simulink model "Impulse_response_system"  (R2022b)
settings: Solver=VariableStepAuto  StartTime=0  StopTime=Tend  FixedStep=0.01  MaxStep=0.1  RelTol=1  AbsTol=1
values from neighbouring files (symbols this model uses):
  I_conversione = Paz.I_conversione    [Glucose_insuline_response.m]    (also in Insulin_controller.m; patient_generator.m = conc_insulina_litro_plasma_Kg)
  IIRb = u(3)    [G_I_Model.m]    (also in Glucose_insuline_response.m = Paz.IIRb; Insulin_controller.m = Paz.IIRb; patient_generator.m = Bolus_die/2)
  Ipb = Paz.Ipb    [Glucose_insuline_response.m]    (also in patient_generator.m = IIRb/(m2+m4 -(m1*m2)/(m1+m3)))
  Pasti = [0,0,0]    [Glucose_insuline_response.m]    (also in Insulin_controller.m = Pasti0+0.2*(-1+2*rand(3,1)).*Pasti0; patient_generator.m = Pasti0)
  Tpasti = Tpasti0    [Glucose_insuline_response.m]    (also in Insulin_controller.m = Tpasti0+delta_T)
  x0 = y(end,1:13)'    [Glucose_insuline_response.m]    (also in Insulin_controller.m; patient_generator.m = [Gp Gt Il Ip I1 Id Qsto1 Qsto2 Qgut X Isc1 Isc2 Dstato])
undefined symbols (not defined in the file or in its folder): Paz
settings Model: Creator=federico  LastModifiedBy=federico
settings SolverCC: MaxConsecutiveMinStep=auto
settings DataIOCC: SaveFormat=Array  SignalLoggingSaveFormat=ModelDataLogs  ReturnWorkspaceOutputs=off
settings OptimizationCC: BlockReduction=off  BooleanDataType=off  InitFltsAndDblsToZero=on  LifeSpan=inf
settings DebuggingCC: SaveWithParameterizedLinksMsg=none  UnderspecifiedInitializationDetection=Classic  MergeDetectMultiDrivingBlocksExec=none  SignalResolutionControl=TryResolveAllWithWarning  MultiTaskDSMMsg=warning  MultiTaskCondExecSysMsg=none  UnconnectedInputMsg=warning  UnconnectedOutputMsg=warning  UnconnectedLineMsg=warning  SFUnexpectedBacktrackingDiag=warning  SFNoUnconditionalDefaultTransitionDiag=warning  SFExecutionAtInitializationDiag=none  SFMachineParentedDataDiag=warning  ArithmeticOperatorsInVariantConditions=warning
settings HardwareCC: ProdBitPerPointer=32  ProdBitPerSizeT=32  ProdBitPerPtrDiffT=32  ProdLargestAtomicFloat=None  ProdIntDivRoundTo=Undefined  ProdEndianess=Unspecified  ProdWordSize=32  ProdHWDeviceType=32-bit Generic  TargetUnknown=on
settings ModelReferenceCC: PropagateSignalLabelsOutOfModel=off
settings CodeAppCC: StateflowObjectComments=on
settings GRTTargetCC: TargetFcnLib=ansi_tfl_tmw.mat  TargetLangStandard=C89/C90 (ANSI)  CombineOutputUpdateFcns=off  GRTInterface=on
settings ConfigComp: CovMetricSettings=dw  CovSaveCumulativeToWorkspaceVar=on  CovSaveSingleToWorkspaceVar=on

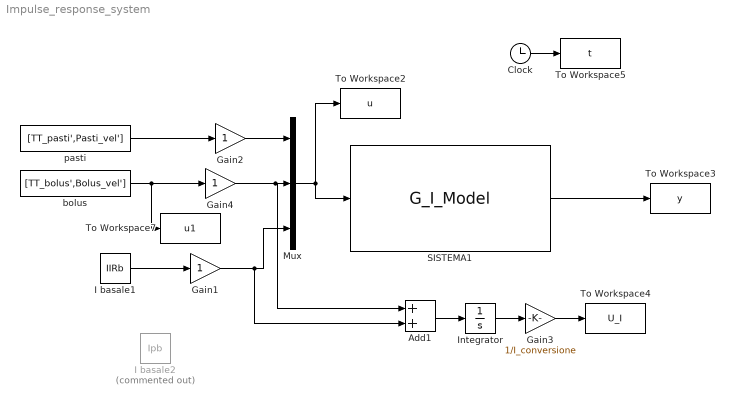
== system Impulse_response_system ==
  Add1 : Sum
  Clock : Clock
  Gain1 : Gain
  Gain2 : Gain
  Gain3 : Gain  Gain=1/I_conversione
  Gain4 : Gain
  I basale1 : Constant  Value=IIRb
  I basale2 : Constant  Commented=on  Value=Ipb
  Integrator : Integrator
  Mux : Mux  Inputs=3
  SISTEMA1 : S-Function  FunctionName=G_I_Model  Parameters=Tpasti,Pasti,Paz,x0  SFunctionDeploymentMode=off  EnableBusSupport=off
  To Workspace2 : ToWorkspace  VariableName=u  SampleTime=1
  To Workspace3 : ToWorkspace  VariableName=y  SampleTime=1
  To Workspace4 : ToWorkspace  VariableName=U_I  SampleTime=1
  To Workspace5 : ToWorkspace  VariableName=t  SampleTime=1
  To Workspace7 : ToWorkspace  VariableName=u1  SampleTime=1
  bolus : FromWorkspace  VariableName=[TT_bolus',Bolus_vel']  ZeroCross=off
  pasti : FromWorkspace  VariableName=[TT_pasti',Pasti_vel']  ZeroCross=off
  wires:
  Clock/1 -> To Workspace5/1
  SISTEMA1/1 -> To Workspace3/1
  Mux/1 -> To Workspace2/1, SISTEMA1/1
  pasti/1 -> Gain2/1
  bolus/1 -> Gain4/1, To Workspace7/1
  Gain2/1 -> Mux/1
  Gain4/1 -> Add1/1, Mux/2
  I basale1/1 -> Gain1/1
  Gain1/1 -> Add1/2, Mux/3
  Integrator/1 -> Gain3/1
  Gain3/1 -> To Workspace4/1
  Add1/1 -> Integrator/1
